simulink model "PID_joint2"  (R2017b)
settings: Solver=VariableStepAuto  StartTime=0.0  StopTime=0.40805  RelTol=1e-3
settings Model: Creator=84935  LastModifiedBy=84935

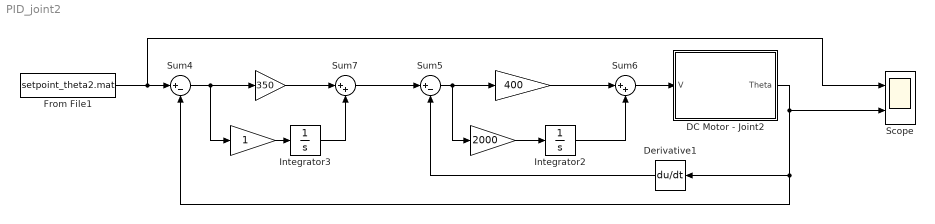
== system PID_joint2 ==
  " " : Gain  Gain=350
  " " : Gain  Gain=2000
  " " : Gain
  " " : Gain  Gain=400
  DC Motor - Joint2 : Subsystem  mask{L=0.012342, R=3.2645, Ki=1.1895, Jeff=0.01829, Beff=0.019, Kb=1.1895, N=100}
  Derivative1 : Derivative
  From File1 : FromFile  FileName=setpoint_theta2.mat  SampleTime=0
  Integrator2 : Integrator
  Integrator3 : Integrator
  Scope : Scope  NumInputPorts=2
  Sum4 : Sum  Inputs=|+-
  Sum5 : Sum  Inputs=|+-
  Sum6 : Sum  Inputs=|++
  Sum7 : Sum  Inputs=|++
  wires:
  Sum6/1 -> DC Motor - Joint2/1(V)
  DC Motor - Joint2/1(Theta) -> Scope/2, Sum4/2, Derivative1/1
  Sum5/1 -> " "/1, " "/1
  Integrator2/1 -> Sum6/2
  " "/1 -> Integrator2/1
  " "/1 -> Sum6/1
  Derivative1/1 -> Sum5/2
  From File1/1 -> Scope/1, Sum4/1
  Integrator3/1 -> Sum7/2
  Sum4/1 -> " "/1, " "/1
  " "/1 -> Sum7/1
  Sum7/1 -> Sum5/1
  " "/1 -> Integrator3/1

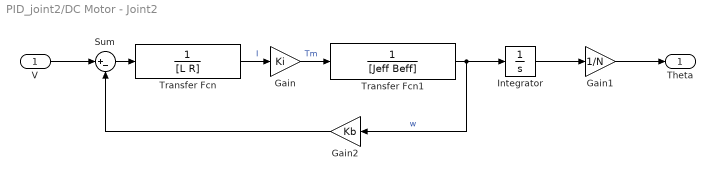
== system PID_joint2/DC Motor - Joint2 ==
  V : Inport
  Gain : Gain  Gain=Ki
  Gain1 : Gain  Gain=1/N
  Gain2 : Gain  Gain=Kb
  Integrator : Integrator
  Sum : Sum  Inputs=|+-
  Transfer Fcn : TransferFcn  Denominator=[L R]
  Transfer Fcn1 : TransferFcn  Denominator=[Jeff Beff]
  Theta : Outport
  wires:
  Integrator/1 -> Gain1/1
  Transfer Fcn1/1 -> Integrator/1, Gain2/1  "w"
  V/1 -> Sum/1
  Gain2/1 -> Sum/2
  Gain/1 -> Transfer Fcn1/1  "Tm"
  Gain1/1 -> Theta/1
  Sum/1 -> Transfer Fcn/1
  Transfer Fcn/1 -> Gain/1  "I"
